simulink model "demostration09"  (R2019b)
settings: Solver=ode45  StartTime=0.0  StopTime=60  RelTol=1e-3  EnableMultiTasking=on
settings Model: Creator=wangze  LastModifiedBy=bhisma
settings DataIOCC: SaveFormat=Array  ReturnWorkspaceOutputs=off
settings OptimizationCC: LifeSpan=inf
settings DebuggingCC: SolverPrmCheckMsg=warning  AllowSymbolicDim=off  SFUnexpectedBacktrackingDiag=warning  SFNoUnconditionalDefaultTransitionDiag=warning  SFExecutionAtInitializationDiag=none  ArithmeticOperatorsInVariantConditions=warning
settings HardwareCC: ProdBitPerPointer=32  ProdBitPerSizeT=32  ProdBitPerPtrDiffT=32  ProdLargestAtomicFloat=None  ProdIntDivRoundTo=Undefined  ProdEndianess=Unspecified  ProdWordSize=32  ProdHWDeviceType=32-bit Generic
settings ModelReferenceCC: PropagateSignalLabelsOutOfModel=off
settings SFSimCC: SimUseLocalCustomCode=off  CustomCodeUndefinedFunction=UseInterfaceOnly
settings RTWCC: RTWUseLocalCustomCode=off
settings CodeAppCC: StateflowObjectComments=on
settings GRTTargetCC: TargetLangStandard=C89/C90 (ANSI)  GeneratePreprocessorConditionals=Disable all
settings ConfigComp: CovMetricSettings=dw  CovHtmlReporting=on  CovSaveCumulativeToWorkspaceVar=on  CovSaveSingleToWorkspaceVar=on  CovExternalEMLEnable=off  CovSFcnEnable=off

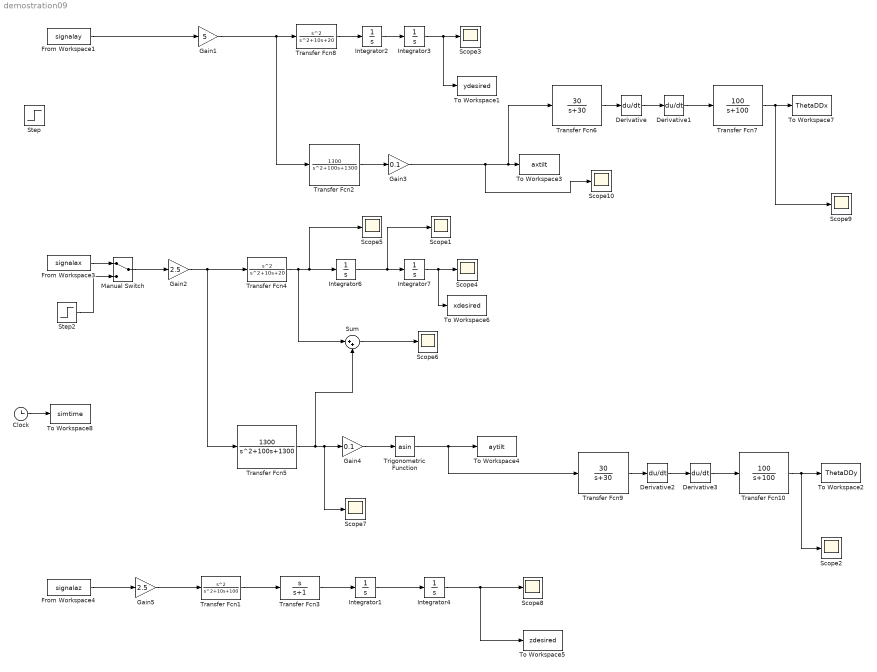
== system demostration09 ==
  Clock : Clock
  Derivative{,1..3} (4 alike) : Derivative  CoefficientInTFapproximation=100
  From Workspace1 : FromWorkspace  VariableName=signalay
  From Workspace3 : FromWorkspace  VariableName=signalax
  From Workspace4 : FromWorkspace  VariableName=signalaz
  Gain1 : Gain  Gain=5  SampleTime=0.05
  Gain2 : Gain  Gain=2.5  SampleTime=0.05
  Gain3 : Gain  Gain=0.1  SampleTime=0.05
  Gain4 : Gain  Gain=0.1  SampleTime=0.05
  Gain5 : Gain  Gain=2.5  SampleTime=0.05
  Integrator{1..4,6..7} (6 alike) : Integrator
  Manual Switch : ManualSwitch
  Scope{1..10} (10 alike) : Scope
  Step : Step  SampleTime=0
  Step2 : Step  Time=0  SampleTime=0
  Sum : Sum  Inputs=|++
  To Workspace1 : ToWorkspace  VariableName=ydesired  SampleTime=-1
      settings: Decimation=2  Save2DSignal=2-D array (concatenate along first dimension)
  To Workspace2 : ToWorkspace  VariableName=ThetaDDy  SampleTime=-1
      settings: Decimation=2
  To Workspace3 : ToWorkspace  VariableName=axtilt  SampleTime=-1
      settings: Decimation=2  Save2DSignal=2-D array (concatenate along first dimension)
  To Workspace4 : ToWorkspace  VariableName=aytilt  SampleTime=-1
      settings: Decimation=2  Save2DSignal=2-D array (concatenate along first dimension)
  To Workspace5 : ToWorkspace  VariableName=zdesired  SampleTime=-1
      settings: Decimation=2
  To Workspace6 : ToWorkspace  VariableName=xdesired  SampleTime=-1
      settings: Decimation=2  Save2DSignal=2-D array (concatenate along first dimension)
  To Workspace7 : ToWorkspace  VariableName=ThetaDDx  SampleTime=-1
      settings: Decimation=2  Save2DSignal=2-D array (concatenate along first dimension)
  To Workspace8 : ToWorkspace  VariableName=simtime  SampleTime=-1
      settings: Decimation=2  Save2DSignal=2-D array (concatenate along first dimension)
  Transfer Fcn1 : TransferFcn  Numerator=[1 0 0]  Denominator=[1 10 100]
  Transfer Fcn10 : TransferFcn  Numerator=[100]  Denominator=[1 100]
  Transfer Fcn2 : TransferFcn  Numerator=[1300]  Denominator=[1 100 1300]
  Transfer Fcn3 : TransferFcn  Numerator=[1 0]  Denominator=[1 1]
  Transfer Fcn4 : TransferFcn  Numerator=[1 0 0]  Denominator=[1 10 20]
  Transfer Fcn5 : TransferFcn  Numerator=[1300]  Denominator=[1 100 1300]
  Transfer Fcn6 : TransferFcn  Numerator=[30]  Denominator=[1 30]
  Transfer Fcn7 : TransferFcn  Numerator=[100]  Denominator=[1 100]
  Transfer Fcn8 : TransferFcn  Numerator=[1 0 0]  Denominator=[1 10 20]
  Transfer Fcn9 : TransferFcn  Numerator=[30]  Denominator=[1 30]
  Trigonometric Function : Trigonometry  Operator=asin
  wires:
  Integrator2/1 -> Integrator3/1
  Integrator3/1 -> Scope3/1, To Workspace1/1
  Integrator6/1 -> Scope1/1, Integrator7/1
  Transfer Fcn4/1 -> Sum/1, Scope5/1, Integrator6/1
  Integrator7/1 -> To Workspace6/1, Scope4/1
  Gain1/1 -> Transfer Fcn2/1, Transfer Fcn8/1
  Gain4/1 -> Trigonometric Function/1
  Transfer Fcn5/1 -> Sum/2, Scope7/1, Gain4/1
  Gain2/1 -> Transfer Fcn5/1, Transfer Fcn4/1
  Manual Switch/1 -> Gain2/1
  From Workspace1/1 -> Gain1/1
  Transfer Fcn8/1 -> Integrator2/1
  From Workspace4/1 -> Gain5/1
  Gain5/1 -> Transfer Fcn1/1
  Transfer Fcn1/1 -> Transfer Fcn3/1
  Transfer Fcn3/1 -> Integrator1/1
  Integrator1/1 -> Integrator4/1
  Integrator4/1 -> To Workspace5/1, Scope8/1
  Step2/1 -> Manual Switch/2
  From Workspace3/1 -> Manual Switch/1
  Sum/1 -> Scope6/1
  Transfer Fcn2/1 -> Gain3/1
  Trigonometric Function/1 -> Transfer Fcn9/1, To Workspace4/1
  Derivative/1 -> Derivative1/1
  Transfer Fcn6/1 -> Derivative/1
  Derivative1/1 -> Transfer Fcn7/1
  Derivative2/1 -> Derivative3/1
  Transfer Fcn9/1 -> Derivative2/1
  Derivative3/1 -> Transfer Fcn10/1
  Transfer Fcn7/1 -> Scope9/1, To Workspace7/1
  Transfer Fcn10/1 -> Scope2/1, To Workspace2/1
  Clock/1 -> To Workspace8/1
  Gain3/1 -> Scope10/1, Transfer Fcn6/1, To Workspace3/1
